simulink model "laser"  (R2017b)
settings: Solver=VariableStepAuto  StartTime=0.0  StopTime=10.0  RelTol=1e-3
values from neighbouring files (symbols this model uses):
  AmpSat1 = NomVoltage    [System.m]
  BackEMF0 = 1/KEmf    [System.m]
  BackEMF1 = 1/KEmf    [System.m]
  Distance = 1    [CONSTANTS.m]
  Elec0d = [La Ra]    [System.m]
  Elec0n = [1]    [System.m]
  Elec1d = [La Ra]    [System.m]
  Elec1n = [1]    [System.m]
  Mech0d = [JSystem KineticFriction 0]    [System.m]
  Mech0n = [1 0]    [System.m]
  Mech1d = [JRotor KineticFriction 0]    [System.m]
  Mech1n = [1 0]    [System.m]
  PWMConversion = [-1.3118e-8 8.6063e-6 -2.0381e-3 0.2134 -0.33242]    [CONSTANTS.m]
  StaticFric = 12e-3    (= 0.012)    [CONSTANTS.m]
  TConst0 = KTorque    [System.m]
  TConst1 = KTorque    [System.m]
undefined symbols (not defined in the file or in its folder): GearRatio, NomI0, NomI1, StallI0, StallI1
libraries: simulink x10
settings Model: Creator=Moochster  LastModifiedBy=lucyl

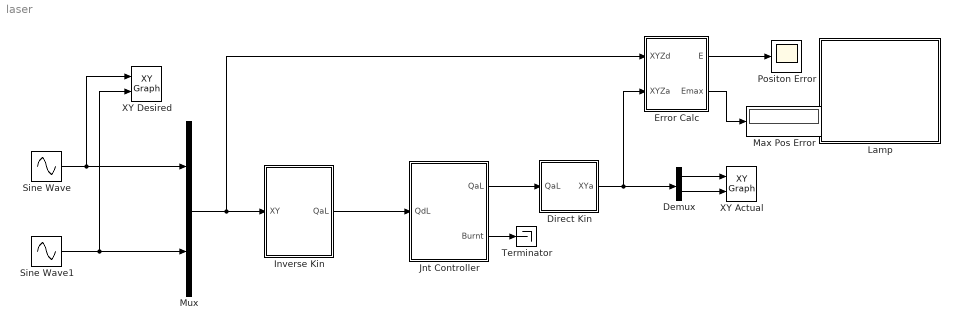
== system laser ==
  Demux : Demux  Outputs=2
  Direct Kin : Subsystem
  Error Calc : Subsystem
  Inverse Kin : Subsystem
  Jnt Controller : Subsystem
  Lamp : Subsystem  DialogController=hmiCreateDDGDialog  IsWebBlock=on  mask(MWDashboardBlock){webBlockId=7fcfd6b5-b98b-441a-9880-35fe4990fbef, webBlockType=lamp, ShowInLibBrowser=on, ShowInitialText=on, HMISrcModelName=laser}
      mask prompts: webBlockType "WebBlock Type"; HMISrcModelName "Source Model"
      mask help: SimulinkHMI:dialogs:LampDialogDesc
      mask Help: helpview([docroot '/mapfiles/simulink.map'], 'hmi_lamp')
      mask Display:
      | if strcmp(get_param(bdroot(gcb),'BlockDiagramType'), 'library')
      |     image([(matlabroot) '/toolbox/simulink/hmi/icons/Lamp.png']);
      | end
  Max Pos Error : Display
  Mux : Mux  Inputs=2
  Positon Error : Scope
  Sine Wave : Sin  Amplitude=50  SampleTime=0
  Sine Wave1 : Sin  Amplitude=50  Phase=pi/2  SampleTime=0
  Terminator : Terminator
  "XY Actual " : simulink/Sinks/XY Graph  xmin=-110  xmax=110  ymin=-110  ymax=110  st=-1
  XY Desired : simulink/Sinks/XY Graph  xmin=-110  xmax=110  ymin=-110  ymax=110  st=-1
  wires:
  Inverse Kin/1(QaL) -> Jnt Controller/1(QdL)
  Jnt Controller/1(QaL) -> Direct Kin/1(QaL)
  Mux/1 -> Error Calc/1(XYZd), Inverse Kin/1(XY)
  Sine Wave/1 -> XY Desired/1, Mux/1
  Sine Wave1/1 -> XY Desired/2, Mux/2
  Demux/2 -> "XY Actual "/2
  Demux/1 -> "XY Actual "/1
  Direct Kin/1(XYa) -> Error Calc/2(XYZa), Demux/1
  Error Calc/1(E) -> Positon Error/1
  Error Calc/2(Emax) -> Max Pos Error/1
  Jnt Controller/2(Burnt) -> Terminator/1

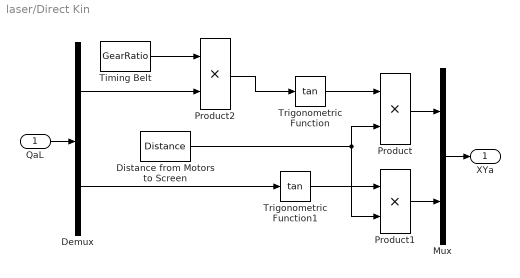
== system laser/Direct Kin ==
  QaL : Inport
  Demux : Demux  Outputs=2
  Distance from Motors to Screen : Constant  Value=Distance
  Mux : Mux  Inputs=2
  Product : Product
  Product1 : Product
  Product2 : Product
  Timing Belt : Constant  Value=GearRatio
  Trigonometric Function : Trigonometry  Operator=tan
  Trigonometric Function1 : Trigonometry  Operator=tan
  XYa : Outport
  wires:
  QaL/1 -> Demux/1
  Mux/1 -> XYa/1
  Demux/1 -> Product2/2
  Demux/2 -> Trigonometric Function1/1
  Trigonometric Function/1 -> Product/1
  Product/1 -> Mux/1
  Product1/1 -> Mux/2
  Trigonometric Function1/1 -> Product1/1
  Distance from Motors to Screen/1 -> Product1/2, Product/2
  Product2/1 -> Trigonometric Function/1
  Timing Belt/1 -> Product2/1

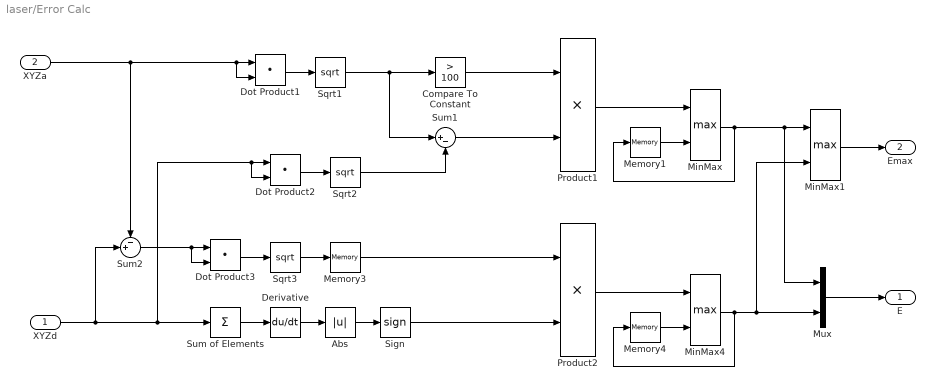
== system laser/Error Calc ==
  XYZd : Inport
  XYZa : Inport  Port=2
  Abs : Abs
  Compare To Constant : simulink/Logic and Bit Operations/Compare To Constant  relop=>  const=100  OutDataTypeStr=boolean
  Derivative : Derivative
  Dot Product1 : DotProduct  InputSameDT=on  OutDataTypeStr=Inherit: Inherit via internal rule
  Dot Product2 : DotProduct  InputSameDT=on  OutDataTypeStr=Inherit: Inherit via internal rule
  Dot Product3 : DotProduct  InputSameDT=on  OutDataTypeStr=Inherit: Inherit via internal rule
  Memory1 : Memory
  Memory3 : Memory
  Memory4 : Memory
  MinMax : MinMax  Function=max  Inputs=2
  MinMax1 : MinMax  Function=max  Inputs=2
  MinMax4 : MinMax  Function=max  Inputs=2
  Mux : Mux  Inputs=2
  Product1 : Product
  Product2 : Product
  Sign : Signum
  Sqrt1 : Sqrt  SaturateOnIntegerOverflow=on
  Sqrt2 : Sqrt  SaturateOnIntegerOverflow=on
  Sqrt3 : Sqrt  SaturateOnIntegerOverflow=on
  Sum of Elements : Sum  Inputs=+
  Sum1 : Sum  Inputs=|+-
  Sum2 : Sum  Inputs=-+|
  E : Outport
  Emax : Outport  Port=2
  wires:
  Sqrt3/1 -> Memory3/1
  Dot Product3/1 -> Sqrt3/1
  Sum2/1 -> Dot Product3/1, Dot Product3/2
  Sqrt2/1 -> Sum1/2
  Dot Product2/1 -> Sqrt2/1
  XYZd/1 -> Dot Product2/1, Dot Product2/2, Sum of Elements/1, Sum2/2
  Memory3/1 -> Product2/1
  Mux/1 -> E/1
  MinMax1/1 -> Emax/1
  MinMax4/1 -> Memory4/1, Mux/2, MinMax1/2
  Product2/1 -> MinMax4/1
  Memory4/1 -> MinMax4/2
  MinMax/1 -> Memory1/1, MinMax1/1, Mux/1
  Memory1/1 -> MinMax/2
  Sum1/1 -> Product1/2
  Compare To Constant/1 -> Product1/1
  Product1/1 -> MinMax/1
  Sqrt1/1 -> Compare To Constant/1, Sum1/1
  Sign/1 -> Product2/2
  Dot Product1/1 -> Sqrt1/1
  XYZa/1 -> Dot Product1/1, Dot Product1/2, Sum2/1
  Sum of Elements/1 -> Derivative/1
  Abs/1 -> Sign/1
  Derivative/1 -> Abs/1

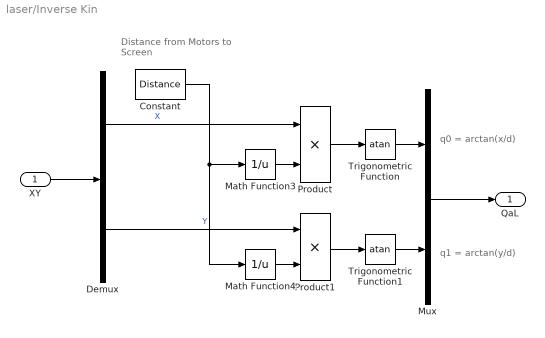
== system laser/Inverse Kin ==
  note: Distance from Motors to Screen
  note: q0 = arctan(x/d)
  note: q1 = arctan(y/d)
  XY : Inport
  Constant : Constant  Value=Distance
  Demux : Demux  Outputs=2
  Math Function3 : Math  Operator=reciprocal  SaturateOnIntegerOverflow=on
  Math Function4 : Math  Operator=reciprocal  SaturateOnIntegerOverflow=on
  Mux : Mux  Inputs=2
  Product : Product
  Product1 : Product
  Trigonometric Function : Trigonometry  Operator=atan
  Trigonometric Function1 : Trigonometry  Operator=atan
  QaL : Outport
  wires:
  XY/1 -> Demux/1
  Mux/1 -> QaL/1
  Demux/1 -> Product/1  "X"
  Demux/2 -> Product1/1  "Y"
  Trigonometric Function/1 -> Mux/1
  Trigonometric Function1/1 -> Mux/2
  Product/1 -> Trigonometric Function/1
  Product1/1 -> Trigonometric Function1/1
  Math Function3/1 -> Product/2
  Math Function4/1 -> Product1/2
  Constant/1 -> Math Function3/1, Math Function4/1

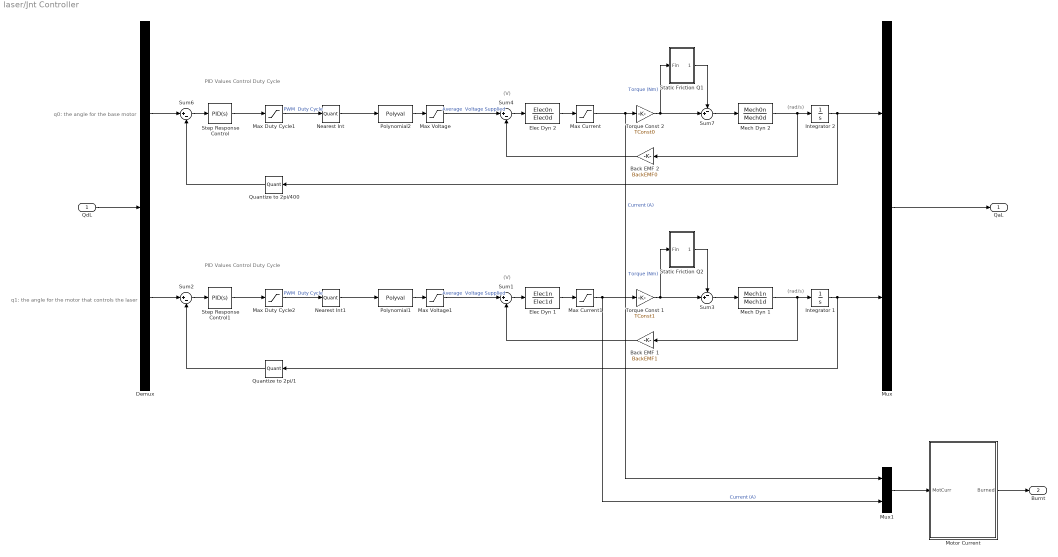
== system laser/Jnt Controller ==
  note: q0: the angle for the base motor
  note: q1: the angle for the motor that controls the laser
  note: (rad/s)
  note: (V)
  note: PID Values Control Duty Cycle
  note: (rad/s)
  note: (V)
  note: PID Values Control Duty Cycle
  QdL : Inport
  Back EMF 1 : Gain  Gain=BackEMF1
  Back EMF 2 : Gain  Gain=BackEMF0
  Demux : Demux  Outputs=2
  Elec Dyn 1 : TransferFcn  Numerator=Elec1n  Denominator=Elec1d
  Elec Dyn 2 : TransferFcn  Numerator=Elec0n  Denominator=Elec0d
  Integrator 1 : Integrator
  Integrator 2 : Integrator
  Max Current : Saturate  UpperLimit=1  LowerLimit=-1
  Max Current1 : Saturate  UpperLimit=1  LowerLimit=-1
  Max Duty Cycle1 : Saturate  UpperLimit=255  LowerLimit=-255
  Max Duty Cycle2 : Saturate  UpperLimit=255  LowerLimit=-255
  Max Voltage : Saturate  UpperLimit=AmpSat1  LowerLimit=-AmpSat1
  Max Voltage1 : Saturate  UpperLimit=AmpSat1  LowerLimit=-AmpSat1
  Mech Dyn 1 : TransferFcn  Numerator=Mech1n  Denominator=Mech1d
  Mech Dyn 2 : TransferFcn  Numerator=Mech0n  Denominator=Mech0d
  Motor Current : Subsystem
  Mux : Mux  Inputs=2
  Mux1 : Mux  Inputs=2
  Nearest Int : Quantizer  QuantizationInterval=1
  Nearest Int1 : Quantizer  QuantizationInterval=1
  Polynomial1 : Polyval  Coefs=PWMConversion
  Polynomial2 : Polyval  Coefs=PWMConversion
  Quantize to 2pi/1 : Quantizer  QuantizationInterval=2*pi/400
  Quantize to 2pi/400 : Quantizer  QuantizationInterval=2*pi/400
  Static Friction Q1 : Subsystem
  Static Friction Q2 : Subsystem
  Step Response Control : simulink/Continuous/PID Controller  Controller=PID  TimeDomain=Continuous-time  SampleTime=-1  IntegratorMethod=Forward Euler  FilterMethod=Forward Euler  Form=Parallel  UseFilter=on  ControllerParametersSource=internal  P=10/pi  I=0  D=0  N=12783.9693192408  InitialConditionSource=internal  InitialConditionForIntegrator=0  InitialConditionForFilter=0  ExternalReset=none  LimitOutput=off  UpperSaturationLimit=inf  LowerSaturationLimit=-inf  LinearizeAsGain=on  AntiWindupMode=none  Kb=1  TrackingMode=off  Kt=1  PParamMin=[]  PParamMax=[]  IParamMin=[]  IParamMax=[]  DParamMin=[]  DParamMax=[]  NParamMin=[]  NParamMax=[]  KbParamMin=[]  KbParamMax=[]  KtParamMin=[]  KtParamMax=[]  POutMin=[]  POutMax=[]  IOutMin=[]  IOutMax=[]  DOutMin=[]  DOutMax=[]  NOutMin=[]  NOutMax=[]  KbOutMin=[]  KbOutMax=[]  KtOutMin=[]  KtOutMax=[]  IntegratorOutMin=[]  IntegratorOutMax=[]  FilterOutMin=[]  FilterOutMax=[]  SumOutMin=[]  SumOutMax=[]  SumI1OutMin=[]  SumI1OutMax=[]  SumI2OutMin=[]  SumI2OutMax=[]  SumI3OutMin=[]  SumI3OutMax=[]  SumDOutMin=[]  SumDOutMax=[]  SaturationOutMin=[]  SaturationOutMax=[]  IntegratorContinuousStateAttributes=''  IntegratorStateMustResolveToSignalObject=off  IntegratorRTWStateStorageClass=Auto  FilterContinuousStateAttributes=''  FilterStateMustResolveToSignalObject=off  FilterRTWStateStorageClass=Auto  DifferentiatorICPrevScaledInput=0  DifferentiatorOutMin=[]  DifferentiatorOutMax=[]  InitialConditionSetting=State (most efficient)  FilterDiffOutCoefMin=[]  FilterDiffOutCoefMax=[]  SumDenOutMin=[]  SumDenOutMax=[]  SumNumOutMin=[]  SumNumOutMax=[]  ReciprocalOutMin=[]  ReciprocalOutMax=[]  DivideOutMin=[]  DivideOutMax=[]  TunerSelectOption=Transfer Function Based (PID Tuner App)
  Step Response Control1 : simulink/Continuous/PID Controller  Controller=PID  TimeDomain=Continuous-time  SampleTime=-1  IntegratorMethod=Forward Euler  FilterMethod=Forward Euler  Form=Parallel  UseFilter=on  ControllerParametersSource=internal  P=10/pi  I=0  D=0  N=12783.9693192408  InitialConditionSource=internal  InitialConditionForIntegrator=0  InitialConditionForFilter=0  ExternalReset=none  LimitOutput=off  UpperSaturationLimit=inf  LowerSaturationLimit=-inf  LinearizeAsGain=on  AntiWindupMode=none  Kb=1  TrackingMode=off  Kt=1  PParamMin=[]  PParamMax=[]  IParamMin=[]  IParamMax=[]  DParamMin=[]  DParamMax=[]  NParamMin=[]  NParamMax=[]  KbParamMin=[]  KbParamMax=[]  KtParamMin=[]  KtParamMax=[]  POutMin=[]  POutMax=[]  IOutMin=[]  IOutMax=[]  DOutMin=[]  DOutMax=[]  NOutMin=[]  NOutMax=[]  KbOutMin=[]  KbOutMax=[]  KtOutMin=[]  KtOutMax=[]  IntegratorOutMin=[]  IntegratorOutMax=[]  FilterOutMin=[]  FilterOutMax=[]  SumOutMin=[]  SumOutMax=[]  SumI1OutMin=[]  SumI1OutMax=[]  SumI2OutMin=[]  SumI2OutMax=[]  SumI3OutMin=[]  SumI3OutMax=[]  SumDOutMin=[]  SumDOutMax=[]  SaturationOutMin=[]  SaturationOutMax=[]  IntegratorContinuousStateAttributes=''  IntegratorStateMustResolveToSignalObject=off  IntegratorRTWStateStorageClass=Auto  FilterContinuousStateAttributes=''  FilterStateMustResolveToSignalObject=off  FilterRTWStateStorageClass=Auto  DifferentiatorICPrevScaledInput=0  DifferentiatorOutMin=[]  DifferentiatorOutMax=[]  InitialConditionSetting=State (most efficient)  FilterDiffOutCoefMin=[]  FilterDiffOutCoefMax=[]  SumDenOutMin=[]  SumDenOutMax=[]  SumNumOutMin=[]  SumNumOutMax=[]  ReciprocalOutMin=[]  ReciprocalOutMax=[]  DivideOutMin=[]  DivideOutMax=[]  TunerSelectOption=Transfer Function Based (PID Tuner App)
  Sum{1..2,4,6} (4 alike) : Sum  Inputs=|+-
  Sum3 : Sum  Inputs=-+|
  Sum7 : Sum  Inputs=-+|
  Torque Const 1 : Gain  Gain=TConst1
  Torque Const 2 : Gain  Gain=TConst0
  QaL : Outport
  Burnt : Outport  Port=2
  wires:
  QdL/1 -> Demux/1
  Demux/1 -> Sum6/1
  Mux/1 -> QaL/1
  Mux1/1 -> Motor Current/1(MotCurr)
  Motor Current/1(Burned) -> Burnt/1
  Static Friction Q1/1(Fout) -> Sum7/1
  Integrator 2/1 -> Mux/1, Quantize to 2pi/400/1
  Nearest Int/1 -> Polynomial2/1
  Torque Const 2/1 -> Sum7/2, Static Friction Q1/1(Fin)  "Torque (Nm)"
  Mech Dyn 2/1 -> Integrator 2/1, Back EMF 2/1
  Sum7/1 -> Mech Dyn 2/1
  Quantize to 2pi/400/1 -> Sum6/2
  Max Current/1 -> Mux1/1, Torque Const 2/1  "Current (A)"
  Polynomial2/1 -> Max Voltage/1
  Step Response Control/1 -> Max Duty Cycle1/1
  Sum4/1 -> Elec Dyn 2/1
  Sum6/1 -> Step Response Control/1
  Elec Dyn 2/1 -> Max Current/1
  Back EMF 2/1 -> Sum4/2
  Max Voltage/1 -> Sum4/1  "Average  Voltage Supplied"
  Max Duty Cycle1/1 -> Nearest Int/1  "PWM  Duty Cycle"
  Max Duty Cycle2/1 -> Nearest Int1/1  "PWM  Duty Cycle"
  Max Voltage1/1 -> Sum1/1  "Average  Voltage Supplied"
  Back EMF 1/1 -> Sum1/2
  Elec Dyn 1/1 -> Max Current1/1
  Sum2/1 -> Step Response Control1/1
  Sum1/1 -> Elec Dyn 1/1
  Step Response Control1/1 -> Max Duty Cycle2/1
  Polynomial1/1 -> Max Voltage1/1
  Max Current1/1 -> Mux1/2, Torque Const 1/1  "Current (A)"
  Quantize to 2pi/1/1 -> Sum2/2
  Sum3/1 -> Mech Dyn 1/1
  Mech Dyn 1/1 -> Back EMF 1/1, Integrator 1/1
  Torque Const 1/1 -> Static Friction Q2/1(Fin), Sum3/2  "Torque (Nm)"
  Nearest Int1/1 -> Polynomial1/1
  Integrator 1/1 -> Mux/2, Quantize to 2pi/1/1
  Static Friction Q2/1(Fout) -> Sum3/1
  Demux/2 -> Sum2/1

== system laser/Lamp ==

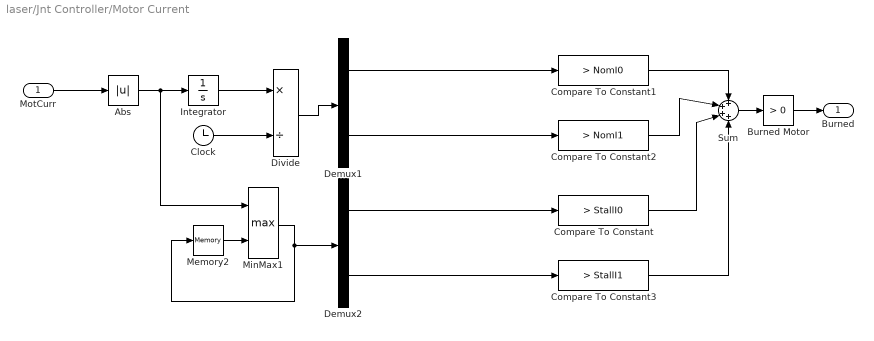
== system laser/Jnt Controller/Motor Current ==
  MotCurr : Inport
  Abs : Abs
  Burned Motor : simulink/Logic and Bit Operations/Compare To Zero  relop=>  OutDataTypeStr=boolean
  Clock : Clock
  Compare To Constant : simulink/Logic and Bit Operations/Compare To Constant  relop=>  const=StallI0  OutDataTypeStr=boolean
  Compare To Constant1 : simulink/Logic and Bit Operations/Compare To Constant  relop=>  const=NomI0  OutDataTypeStr=boolean
  Compare To Constant2 : simulink/Logic and Bit Operations/Compare To Constant  relop=>  const=NomI1  OutDataTypeStr=boolean
  Compare To Constant3 : simulink/Logic and Bit Operations/Compare To Constant  relop=>  const=StallI1  OutDataTypeStr=boolean
  Demux1 : Demux  Outputs=2
  Demux2 : Demux  Outputs=2
  Divide : Product  Inputs=*/
  Integrator : Integrator
  Memory2 : Memory
  MinMax1 : MinMax  Function=max  Inputs=2
  Sum : Sum  Inputs=++++
  Burned : Outport
  wires:
  Sum/1 -> Burned Motor/1
  Burned Motor/1 -> Burned/1
  MinMax1/1 -> Memory2/1, Demux2/1
  Memory2/1 -> MinMax1/2
  Compare To Constant2/1 -> Sum/2
  Compare To Constant/1 -> Sum/3
  Compare To Constant3/1 -> Sum/4
  Compare To Constant1/1 -> Sum/1
  Demux2/2 -> Compare To Constant3/1
  Demux1/2 -> Compare To Constant2/1
  Demux2/1 -> Compare To Constant/1
  Abs/1 -> Integrator/1, MinMax1/1
  Divide/1 -> Demux1/1
  Clock/1 -> Divide/2
  Integrator/1 -> Divide/1
  MotCurr/1 -> Abs/1
  Demux1/1 -> Compare To Constant1/1

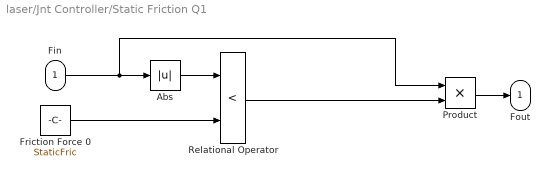
== system laser/Jnt Controller/Static Friction Q1 ==
  Fin : Inport
  Abs : Abs
  Friction Force 0 : Constant  Value=StaticFric
  Product : Product
  Relational Operator : RelationalOperator  Operator=<  OutDataTypeStr=boolean  RndMeth=Simplest
  Fout : Outport
  wires:
  Relational Operator/1 -> Product/2
  Friction Force 0/1 -> Relational Operator/2
  Product/1 -> Fout/1
  Fin/1 -> Abs/1, Product/1
  Abs/1 -> Relational Operator/1

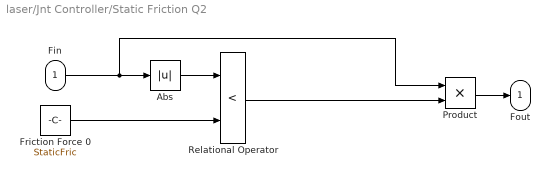
== system laser/Jnt Controller/Static Friction Q2 ==
  Fin : Inport
  Abs : Abs
  Friction Force 0 : Constant  Value=StaticFric
  Product : Product
  Relational Operator : RelationalOperator  Operator=<  OutDataTypeStr=boolean  RndMeth=Simplest
  Fout : Outport
  wires:
  Abs/1 -> Relational Operator/1
  Fin/1 -> Product/1, Abs/1
  Product/1 -> Fout/1
  Friction Force 0/1 -> Relational Operator/2
  Relational Operator/1 -> Product/2
